simulink model "a4"  (R2020a)
settings: Solver=VariableStepAuto  StartTime=0.0  StopTime=15  RelTol=1e-3
undefined symbols (not defined in the file): sigbuilder_block
settings Model: Creator=bill2  LastModifiedBy=bill2
settings DataIOCC: Refine=10

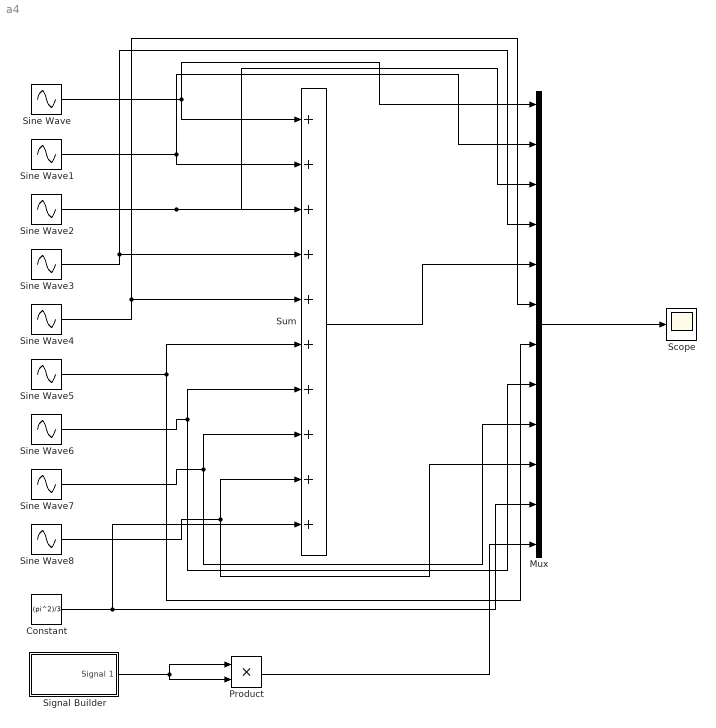
== system a4 ==
  Constant : Constant  Value=(pi^2)/3
  Mux : Mux  Inputs=12
  Product : Product
  Scope : Scope
  Signal Builder : Subsystem  Tag=STV Subsys  LoadFcn=sigbuilder_block('load');  StartFcn=sigbuilder_block('start');  StopFcn=sigbuilder_block('stop');  ClipboardFcn=sigbuilder_block('clipboard');  mask(Sigbuilder block){tuvar=[0:10]}
      mask help: Simulink:masks:SigbuilderBlock_MD
      mask init:
      | if ~strcmp(get_param(bdroot(gcbh),'SimulationStatus'),'stopped') tuvar = sigbuilder_block('maskInit'); end
      settings: CopyFcn=sigbuilder_block('copy');  DeleteFcn=sigbuilder_block('delete');  ModelCloseFcn=sigbuilder_block('modelClose');  PreSaveFcn=sigbuilder_block('preSave');  PauseFcn=sigbuilder_block('pause');  ContinueFcn=sigbuilder_block('continue');  NameChangeFcn=sigbuilder_block('namechange');  OpenFcn=sigbuilder_block('open',[437.6 199.2 550.4 400 ]);  CloseFcn=sigbuilder_block('close');
      mask Display: plot(0, 0, 100, 100,[2, 2, 32, 32, 2], [68, 8, 8, 68, 68],[32, 2], [38, 38], [32, 19, 2],[53, 60, 44], [32, 17, 17, 2],[16, 16, 31, 31]);txt = getActiveGroup(gcbh);text(2, 100, txt,'verticalAlignment', 'top');
  Sine Wave : Sin  Amplitude=-4  Phase=pi/2  SampleTime=0
  Sine Wave1 : Sin  Frequency=2  Phase=pi/2  SampleTime=0
  Sine Wave2 : Sin  Amplitude=-4/9  Frequency=3  Phase=pi/2  SampleTime=0
  Sine Wave3 : Sin  Amplitude=1/4  Frequency=4  Phase=pi/2  SampleTime=0
  Sine Wave4 : Sin  Amplitude=-4/25  Frequency=5  Phase=pi/2  SampleTime=0
  Sine Wave5 : Sin  Amplitude=4/36  Frequency=6  Phase=pi/2  SampleTime=0
  Sine Wave6 : Sin  Amplitude=-4/49  Frequency=7  Phase=pi/2  SampleTime=0
  Sine Wave7 : Sin  Amplitude=4/64  Frequency=8  Phase=pi/2  SampleTime=0
  Sine Wave8 : Sin  Amplitude=-4/81  Frequency=9  Phase=pi/2  SampleTime=0
  Sum : Sum  Inputs=10
  wires:
  Sine Wave/1 -> Mux/1, Sum/1
  Sine Wave1/1 -> Mux/2, Sum/2
  Sine Wave2/1 -> Mux/3, Sum/3
  Sine Wave3/1 -> Mux/4, Sum/4
  Sine Wave4/1 -> Mux/6, Sum/5
  Sine Wave5/1 -> Mux/7, Sum/6
  Sine Wave6/1 -> Mux/8, Sum/7
  Sine Wave7/1 -> Mux/9, Sum/8
  Sine Wave8/1 -> Mux/10, Sum/9
  Sum/1 -> Mux/5
  Constant/1 -> Sum/10, Mux/11
  Signal Builder/1(Signal 1) -> Product/2, Product/1
  Mux/1 -> Scope/1
  Product/1 -> Mux/12

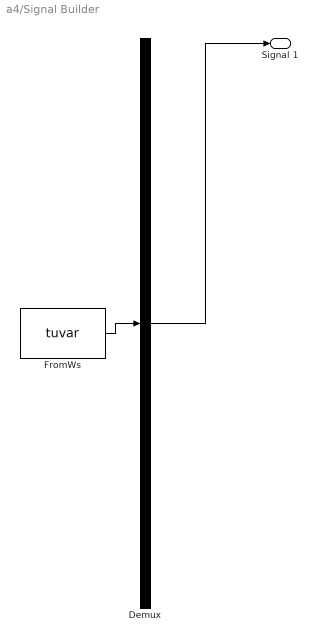
== system a4/Signal Builder ==
  Demux : Demux  Tag=STV Demux  Outputs=1
      settings: DisplayOption=none
  FromWs : FromWorkspace  Tag=STV FromWs  VariableName=tuvar
      SigBuilderData=|
      | common.afterFinalStr = 'Extrapolate'
      | common.sampleTime = 0
      | dataSet.timeRange = [0 18.8495559215]
      | dataSet.name = 'Group 1'
      | sbobj.Groups.Name = 'Group 1'
      | sbobj.Groups.Signals.Name = 'Signal 1'
      | sbobj.Groups.Signals.XData = [0 3.14159265359 6.28318530718 9.42477796077 12.5663706144 15.7079632679 18.8495559215]
      | sbobj.Groups.Signals.YData = [0 3.14159265359 0 3.14159265359 0 3.14159265359 0]
      | sbobj.Groups.TimeRange = [0 18.8495559215]
  Signal 1 : Outport  Tag=STV Outport
  wires:
  Demux/1 -> Signal 1/1
  FromWs/1 -> Demux/1
